simulink model "Version7_twogyros_nl"  (R2019a)
settings: Solver=VariableStepAuto  StartTime=0.0  StopTime=10  RelTol=1e-3
values from neighbouring files (symbols this model uses):
  Dist_period = 10    [LQR_PLACE_v9_sep_gryos.m]
  F_d = 11    [LQR_PLACE_v9_sep_gryos.m]
  Fd = 600    [LQR_PLACE_v9_sep_gryos.m]
  g = 9.81    [LQR_PLACE_v9_sep_gryos.m]
  hb = 0.21311    [LQR_PLACE_v9_sep_gryos.m]
  Igz = 0.062    [LQR_PLACE_v9_sep_gryos.m]
  init_roll_angle = pi/180*15    (= 0.261799387799)    [LQR_PLACE_v9_sep_gryos.m]
  init_roll_rate = 0    [LQR_PLACE_v9_sep_gryos.m]
  k1 = Icx + Igx    (= 0.132)    [LQR_PLACE_v9_sep_gryos.m]
  k2 = Icy + Igy    (= 0.146)    [LQR_PLACE_v9_sep_gryos.m]
  k3 = Icz + Igz    (= 0.216)    [LQR_PLACE_v9_sep_gryos.m]
  k4 = Ibx + 2*Isx    (= 10.856)    [LQR_PLACE_v9_sep_gryos.m]
  k5 = k1 - k3    (= -0.084)    [LQR_PLACE_v9_sep_gryos.m]
  k6 = 2*hg*( mc + mg ) + hb*mb + 2*hs*ms    (= 30.78237461)    [LQR_PLACE_v9_sep_gryos.m]
  k7 = 2*( hg^2 )*( mc + mg ) + ( hb^2 )*mb + 2*( hs^2 )*ms    (= 6.80796014274)    [LQR_PLACE_v9_sep_gryos.m]
  omega1 = 536.6    [LQR_PLACE_v9_sep_gryos.m]
  omega2 = -536.6    [LQR_PLACE_v9_sep_gryos.m]
  Ts = Ts_min    [LQR_PLACE_v9_sep_gryos.m]
undefined symbols (not defined in the file or in its folder): Kd
libraries: simulink_extras x3
settings Model: Creator=nziv  LastModifiedBy=nata9
settings DebuggingCC: ArithmeticOperatorsInVariantConditions=warning

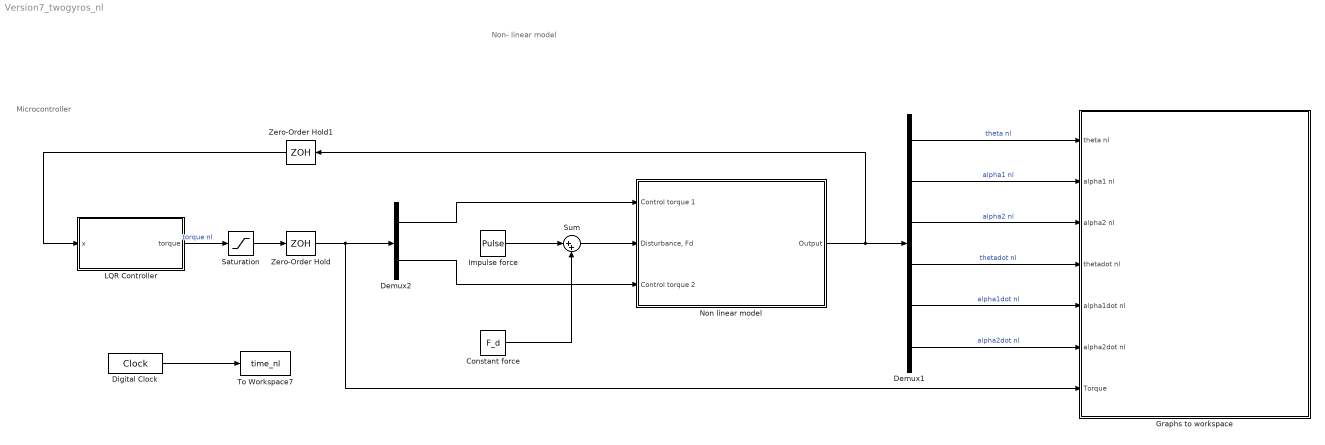
== system Version7_twogyros_nl ==
  note: Microcontroller
  note: Non- linear model
  "Constant force " : Constant  Value=F_d
  Demux1 : Demux  Outputs=6
  Demux2 : Demux  Outputs=2
  Digital Clock : DigitalClock  SampleTime=Ts
  "Graphs to workspace " : Subsystem
  "Impulse force " : DiscretePulseGenerator  PulseType=Time based  Amplitude=Fd  Period=Dist_period  PulseWidth=5  PhaseDelay=5
  LQR Controller : Subsystem
  Non linear model : Subsystem
  Saturation : Saturate  UpperLimit=70  LowerLimit=-70
  Sum : Sum  Inputs=|++
  To Workspace7 : ToWorkspace  VariableName=time_nl  SampleTime=-1
  Zero-Order Hold : ZeroOrderHold  SampleTime=Ts
  Zero-Order Hold1 : ZeroOrderHold  SampleTime=Ts
  wires:
  Non linear model/1(Output) -> Demux1/1, Zero-Order Hold1/1
  LQR Controller/1(torque) -> Saturation/1  "torque nl"
  Demux2/1 -> Non linear model/1(Control torque 1)
  Demux2/2 -> Non linear model/3(Control torque 2)
  Zero-Order Hold/1 -> "Graphs to workspace "/7(Torque), Demux2/1
  Zero-Order Hold1/1 -> LQR Controller/1(x)
  Digital Clock/1 -> To Workspace7/1
  Demux1/1 -> "Graphs to workspace "/1(theta nl)  "theta nl"
  Demux1/2 -> "Graphs to workspace "/2(alpha1 nl)  "alpha1 nl"
  Demux1/3 -> "Graphs to workspace "/3(alpha2 nl)  "alpha2 nl"
  Demux1/4 -> "Graphs to workspace "/4(thetadot nl)  "thetadot nl"
  Demux1/5 -> "Graphs to workspace "/5(alpha1dot nl)  "alpha1dot nl"
  Demux1/6 -> "Graphs to workspace "/6(alpha2dot nl)  "alpha2dot nl"
  "Impulse force "/1 -> Sum/1
  Sum/1 -> Non linear model/2("Disturbance, Fd")
  "Constant force "/1 -> Sum/2
  Saturation/1 -> Zero-Order Hold/1

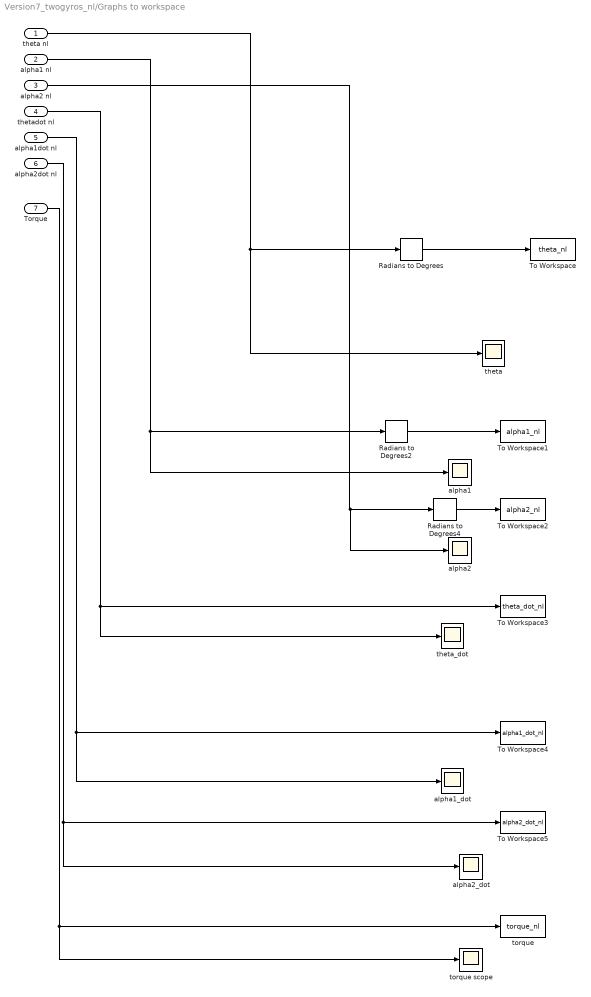
== system Version7_twogyros_nl/Graphs to workspace  ==
  theta nl : Inport
  alpha1 nl : Inport  Port=2
  alpha2 nl : Inport  Port=3
  thetadot nl : Inport  Port=4
  alpha1dot nl : Inport  Port=5
  alpha2dot nl : Inport  Port=6
  Torque : Inport  Port=7
  Radians to Degrees : simulink_extras/Transformations/Radians to Degrees
  Radians to Degrees2 : simulink_extras/Transformations/Radians to Degrees
  Radians to Degrees4 : simulink_extras/Transformations/Radians to Degrees
  To Workspace : ToWorkspace  VariableName=theta_nl  SampleTime=Ts
  To Workspace1 : ToWorkspace  VariableName=alpha1_nl  SampleTime=Ts
  To Workspace2 : ToWorkspace  VariableName=alpha2_nl  SampleTime=Ts
  To Workspace3 : ToWorkspace  VariableName=theta_dot_nl  SampleTime=Ts
  To Workspace4 : ToWorkspace  VariableName=alpha1_dot_nl  SampleTime=Ts
  To Workspace5 : ToWorkspace  VariableName=alpha2_dot_nl  SampleTime=Ts
  alpha1 : Scope
  alpha1_dot : Scope
  alpha2 : Scope
  alpha2_dot : Scope
  theta : Scope
  theta_dot : Scope
  torque : ToWorkspace  VariableName=torque_nl  SampleTime=Ts
  torque scope : Scope
  wires:
  Radians to Degrees4/1 -> To Workspace2/1
  alpha1 nl/1 -> alpha1/1, Radians to Degrees2/1
  alpha1dot nl/1 -> alpha1_dot/1, To Workspace4/1
  alpha2 nl/1 -> alpha2/1, Radians to Degrees4/1
  theta nl/1 -> theta/1, Radians to Degrees/1
  Radians to Degrees/1 -> To Workspace/1
  Radians to Degrees2/1 -> To Workspace1/1
  thetadot nl/1 -> theta_dot/1, To Workspace3/1
  alpha2dot nl/1 -> alpha2_dot/1, To Workspace5/1
  Torque/1 -> torque/1, torque scope/1

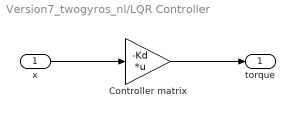
== system Version7_twogyros_nl/LQR Controller ==
  x : Inport
  Controller matrix : Gain  Gain=-Kd  Multiplication=Matrix(K*u)
  torque : Outport
  wires:
  Controller matrix/1 -> torque/1
  x/1 -> Controller matrix/1

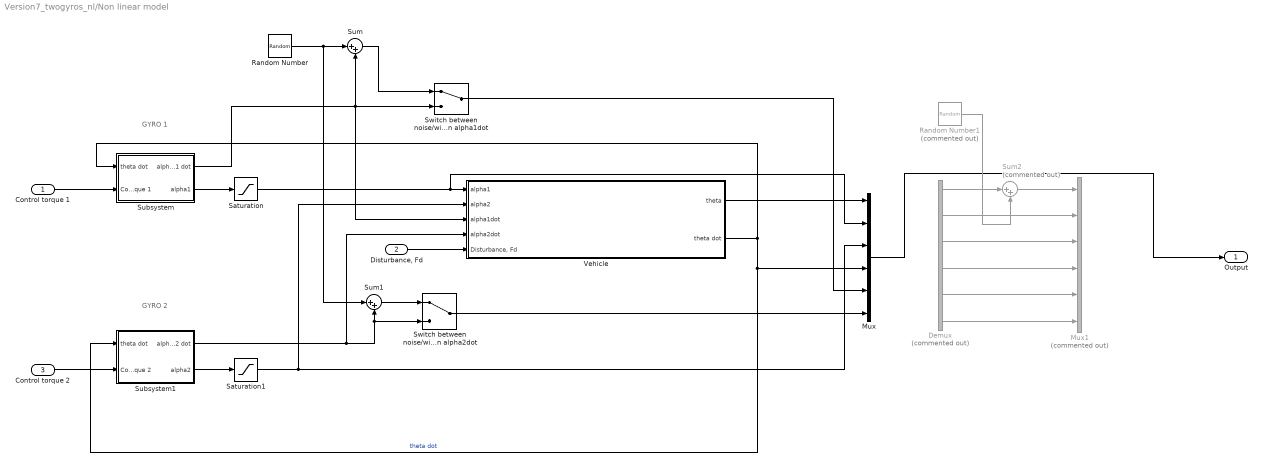
== system Version7_twogyros_nl/Non linear model ==
  note: GYRO 2
  note: GYRO 1
  Control torque 1 : Inport
  "Disturbance, Fd" : Inport  Port=2
  Control torque 2 : Inport  Port=3
  Demux : Demux  Commented=on  Outputs=6
  Mux : Mux  Inputs=6
  Mux1 : Mux  Commented=on  Inputs=6
  Random Number : RandomNumber  Variance=0.01  Seed=34567  SampleTime=Ts
  Random Number1 : RandomNumber  Commented=on  Variance=0.00001  Seed=23456  SampleTime=Ts
  Saturation : Saturate  UpperLimit=(50*pi)/180  LowerLimit=-(50*pi)/180
  Saturation1 : Saturate  UpperLimit=(50*pi)/180  LowerLimit=-(50*pi)/180
  Subsystem : Subsystem
  Subsystem1 : Subsystem
  Sum : Sum  Inputs=|++
  Sum1 : Sum  Inputs=|++
  Sum2 : Sum  Commented=on  Inputs=|++
  Switch between noise/without noise on alpha1dot : ManualSwitch
  Switch between noise/without noise on alpha2dot : ManualSwitch
  "Vehicle " : Subsystem
  Output : Outport
  wires:
  "Vehicle "/2(theta dot) -> Mux/4, Subsystem1/1(theta dot), Subsystem/1(theta dot)  "theta dot"
  "Disturbance, Fd"/1 -> "Vehicle "/5("Disturbance, Fd")
  Subsystem1/2(alpha2) -> Saturation1/1
  Control torque 1/1 -> Subsystem/2(Control torque 1)
  Subsystem/2(alpha1) -> Saturation/1
  Control torque 2/1 -> Subsystem1/2(Control torque 2)
  Random Number/1 -> Sum/1, Sum1/1
  Subsystem1/1(alpha2 dot) -> Switch between noise/without noise on alpha2dot/2, Sum1/2, "Vehicle "/4(alpha2dot)
  Subsystem/1(alpha1 dot) -> "Vehicle "/3(alpha1dot), Switch between noise/without noise on alpha1dot/2, Sum/2
  Sum/1 -> Switch between noise/without noise on alpha1dot/1
  Sum1/1 -> Switch between noise/without noise on alpha2dot/1
  Switch between noise/without noise on alpha1dot/1 -> Mux/5
  "Vehicle "/1(theta) -> Mux/1
  Saturation/1 -> Mux/2, "Vehicle "/1(alpha1)
  Saturation1/1 -> Mux/3, "Vehicle "/2(alpha2)
  Switch between noise/without noise on alpha2dot/1 -> Mux/6
  Mux/1 -> Output/1
  Demux/6 -> Mux1/6
  Demux/5 -> Mux1/5
  Demux/4 -> Mux1/4
  Demux/3 -> Mux1/3
  Demux/2 -> Mux1/2
  Demux/1 -> Sum2/1
  Sum2/1 -> Mux1/1
  Random Number1/1 -> Sum2/2

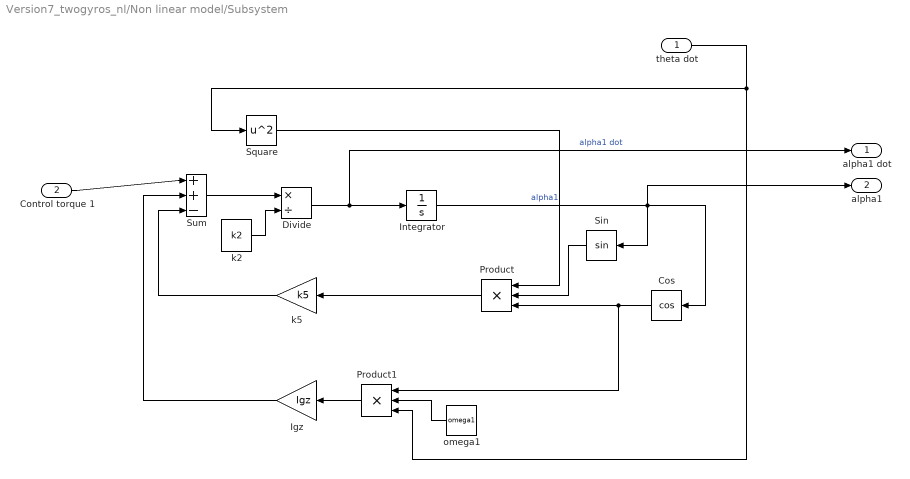
== system Version7_twogyros_nl/Non linear model/Subsystem ==
  theta dot : Inport
  Control torque 1 : Inport  Port=2
  Cos : Trigonometry  Operator=cos
  Divide : Product  Inputs=*/
  Igz : Gain  Gain=Igz
  Integrator : Integrator
  Product : Product  Inputs=3
  Product1 : Product  Inputs=3
  Sin : Trigonometry
  Square : Math  Operator=square  SaturateOnIntegerOverflow=on
  Sum : Sum  Inputs=|++-
  k2 : Constant  Value=k2
  k5 : Gain  Gain=k5
  omega1 : Constant  Value=omega1
  alpha1 dot : Outport
  alpha1 : Outport  Port=2
  wires:
  theta dot/1 -> Product1/3, Square/1
  Square/1 -> Product/1
  Cos/1 -> Product/3, Product1/1
  Igz/1 -> Sum/2
  Sin/1 -> Product/2
  omega1/1 -> Product1/2
  Product/1 -> k5/1
  Integrator/1 -> Cos/1, Sin/1, alpha1/1  "alpha1"
  Product1/1 -> Igz/1
  k2/1 -> Divide/2
  Divide/1 -> alpha1 dot/1, Integrator/1  "alpha1 dot"
  Sum/1 -> Divide/1
  k5/1 -> Sum/3
  Control torque 1/1 -> Sum/1

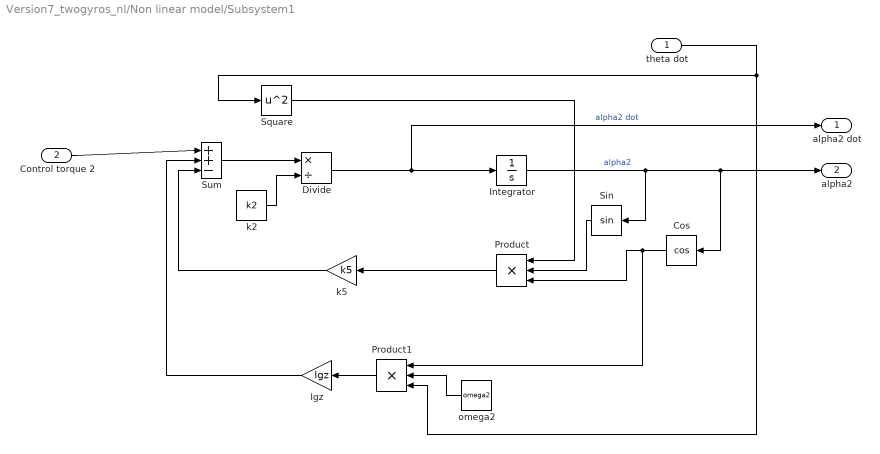
== system Version7_twogyros_nl/Non linear model/Subsystem1 ==
  theta dot : Inport
  Control torque 2 : Inport  Port=2
  Cos : Trigonometry  Operator=cos
  Divide : Product  Inputs=*/
  Igz : Gain  Gain=Igz
  Integrator : Integrator
  Product : Product  Inputs=3
  Product1 : Product  Inputs=3
  Sin : Trigonometry
  Square : Math  Operator=square  SaturateOnIntegerOverflow=on
  Sum : Sum  Inputs=|++-
  k2 : Constant  Value=k2
  k5 : Gain  Gain=k5
  omega2 : Constant  Value=omega2
  alpha2 dot : Outport
  alpha2 : Outport  Port=2
  wires:
  theta dot/1 -> Product1/3, Square/1
  Square/1 -> Product/1
  Cos/1 -> Product/3, Product1/1
  Igz/1 -> Sum/2
  Sin/1 -> Product/2
  omega2/1 -> Product1/2
  Product/1 -> k5/1
  Integrator/1 -> alpha2/1, Cos/1, Sin/1  "alpha2"
  Product1/1 -> Igz/1
  k2/1 -> Divide/2
  Divide/1 -> alpha2 dot/1, Integrator/1  "alpha2 dot"
  Sum/1 -> Divide/1
  k5/1 -> Sum/3
  Control torque 2/1 -> Sum/1

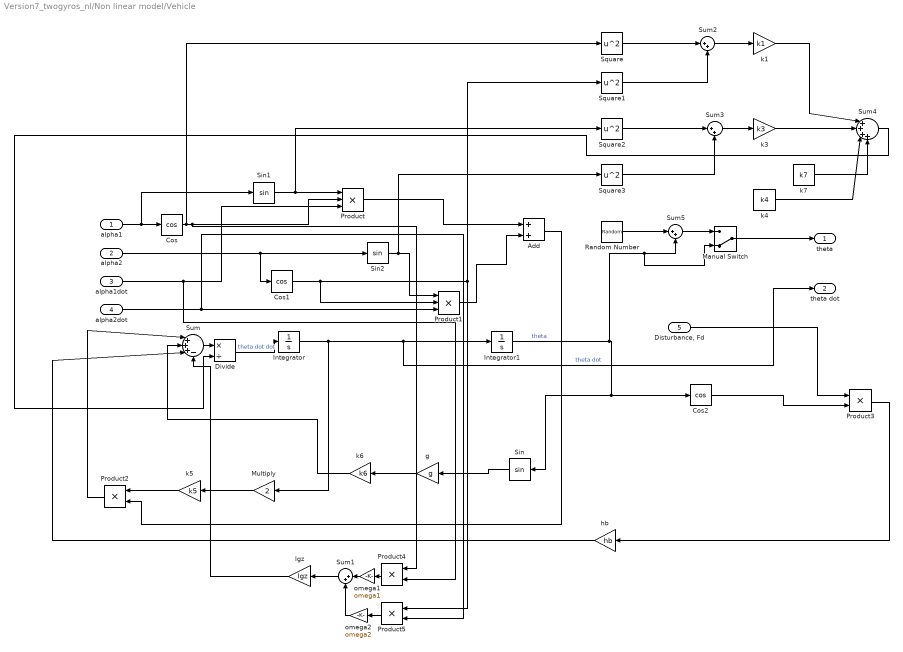
== system Version7_twogyros_nl/Non linear model/Vehicle  ==
  alpha1 : Inport
  alpha2 : Inport  Port=2
  alpha1dot : Inport  Port=3
  alpha2dot : Inport  Port=4
  "Disturbance, Fd" : Inport  Port=5
  Add : Sum
  Cos : Trigonometry  Operator=cos
  Cos1 : Trigonometry  Operator=cos
  Cos2 : Trigonometry  Operator=cos
  Divide : Product  Inputs=*/
  Igz : Gain  Gain=Igz
  Integrator : Integrator  InitialCondition=init_roll_rate
  Integrator1 : Integrator  InitialCondition=init_roll_angle
  Manual Switch : ManualSwitch  CurrentSetting=0
  Multiply : Gain  Gain=2
  Product : Product  Inputs=3
  Product1 : Product  Inputs=3
  Product{2..5} (4 alike) : Product
  Random Number : RandomNumber  Variance=0.01  Seed=34567  SampleTime=0.7
  Sin : Trigonometry
  Sin1 : Trigonometry
  Sin2 : Trigonometry
  Square{,1..3} (4 alike) : Math  Operator=square  SaturateOnIntegerOverflow=on
  Sum : Sum  Inputs=|+++-
  Sum{1..3,5} (4 alike) : Sum  Inputs=|++
  Sum4 : Sum  Inputs=|++++
  g : Gain  Gain=g
  hb : Gain  Gain=hb
  k1 : Gain  Gain=k1
  k3 : Gain  Gain=k3
  k4 : Constant  Value=k4
  k5 : Gain  Gain=k5
  k6 : Gain  Gain=k6
  k7 : Constant  Value=k7
  omega1 : Gain  Gain=omega1
  omega2 : Gain  Gain=omega2
  theta : Outport
  theta dot : Outport  Port=2
  wires:
  Cos/1 -> Square/1, Product4/1, Product/2
  alpha2/1 -> Sin2/1, Cos1/1
  Integrator/1 -> theta dot/1, Integrator1/1, Multiply/1  "theta dot"
  Product/1 -> Add/1
  Sin/1 -> g/1
  Product2/1 -> Sum/1
  k6/1 -> Sum/2
  alpha1dot/1 -> Product4/2, Product/3
  Igz/1 -> Sum/4
  Sin1/1 -> Square2/1, Product/1
  Cos1/1 -> Square1/1, Product5/1, Product1/2
  alpha1/1 -> Sin1/1, Cos/1
  Add/1 -> Product2/2
  alpha2dot/1 -> Product5/2, Product1/3
  Integrator1/1 -> Sin/1, Cos2/1, Manual Switch/2, Sum5/2  "theta"
  g/1 -> k6/1
  hb/1 -> Sum/3
  Product1/1 -> Add/2
  Product4/1 -> omega1/1
  Cos2/1 -> Product3/2
  "Disturbance, Fd"/1 -> Product3/1
  Sin2/1 -> Square3/1, Product1/1
  Product3/1 -> hb/1
  k5/1 -> Product2/1
  Sum1/1 -> Igz/1
  Multiply/1 -> k5/1
  Product5/1 -> omega2/1
  Square/1 -> Sum2/1
  Square1/1 -> Sum2/2
  Sum2/1 -> k1/1
  Square2/1 -> Sum3/1
  Square3/1 -> Sum3/2
  Sum3/1 -> k3/1
  k1/1 -> Sum4/1
  k3/1 -> Sum4/2
  k4/1 -> Sum4/3
  Sum/1 -> Divide/1
  Divide/1 -> Integrator/1  "theta dot dot"
  Sum4/1 -> Divide/2
  k7/1 -> Sum4/4
  omega2/1 -> Sum1/2
  omega1/1 -> Sum1/1
  Random Number/1 -> Sum5/1
  Sum5/1 -> Manual Switch/1
  Manual Switch/1 -> theta/1
